simulink model "Basic_PLL_Beating1"  (R2014a)
settings: Solver=ode45  StartTime=0.0  StopTime=10.0  MaxStep=0.001  RelTol=1e-3
values from neighbouring files (symbols this model uses):
  IC_1 = 0.55    [Run_Basic_PLL_Beating1.m]
  IC_2 = -0.55    [Run_Basic_PLL_Beating1.m]
  Step_size = +0.47    (= 0.47)    [Run_Basic_PLL_Beating1.m]
settings Model: Creator=USER  LastModifiedBy=USER
settings SolverCC: InitialStep=0.001

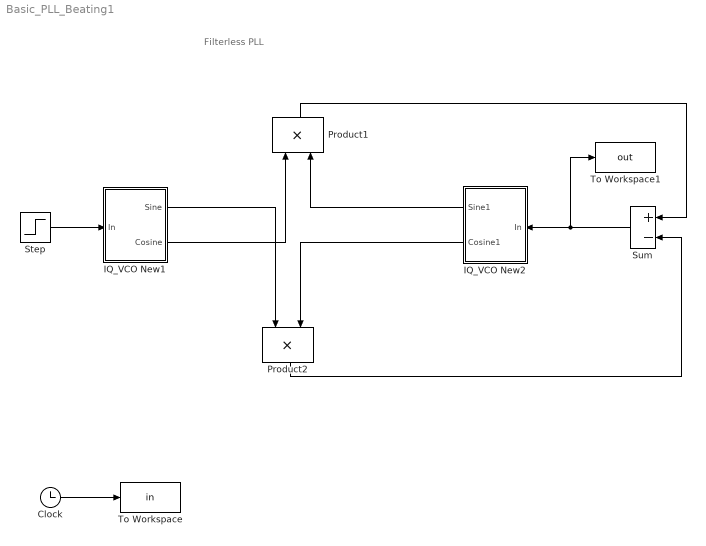
== system Basic_PLL_Beating1 ==
  note: Filterless PLL
  Clock : Clock
  IQ_VCO New1 : Subsystem
  IQ_VCO New2 : Subsystem
  Product1 : Product  SaturateOnIntegerOverflow=on  OutDataTypeStr=Inherit: Same as first input
  Product2 : Product  SaturateOnIntegerOverflow=on  OutDataTypeStr=Inherit: Same as first input
  Step : Step  Time=0  After=Step_size  SampleTime=0
  Sum : Sum  Inputs=+-  SaturateOnIntegerOverflow=on
  To Workspace : ToWorkspace  VariableName=in  SampleTime=-1
  To Workspace1 : ToWorkspace  VariableName=out  SampleTime=-1
  wires:
  Step/1 -> IQ_VCO New1/1(In)
  IQ_VCO New1/2(Cosine) -> Product1/1
  IQ_VCO New2/2(Cosine1) -> Product2/2
  IQ_VCO New1/1(Sine) -> Product2/1
  IQ_VCO New2/1(Sine1) -> Product1/2
  Sum/1 -> To Workspace1/1, IQ_VCO New2/1(In)
  Product1/1 -> Sum/1
  Product2/1 -> Sum/2
  Clock/1 -> To Workspace/1

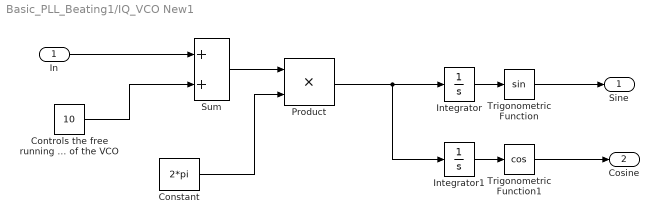
== system Basic_PLL_Beating1/IQ_VCO New1 ==
  In : Inport
  Constant : Constant  Value=2*pi
  "Controls the free running frequency (Hz) of the VCO " : Constant  Value=10
  Integrator : Integrator  InitialCondition=IC_1
  Integrator1 : Integrator  InitialCondition=IC_2
  Product : Product  SaturateOnIntegerOverflow=on  OutDataTypeStr=Inherit: Same as first input
  Sum : Sum  SaturateOnIntegerOverflow=on
  Trigonometric Function : Trigonometry
  Trigonometric Function1 : Trigonometry  Operator=cos
  Sine : Outport
  Cosine : Outport  Port=2
  wires:
  In/1 -> Sum/1
  "Controls the free running frequency (Hz) of the VCO "/1 -> Sum/2
  Sum/1 -> Product/1
  Constant/1 -> Product/2
  Trigonometric Function/1 -> Sine/1
  Trigonometric Function1/1 -> Cosine/1
  Integrator/1 -> Trigonometric Function/1
  Integrator1/1 -> Trigonometric Function1/1
  Product/1 -> Integrator1/1, Integrator/1

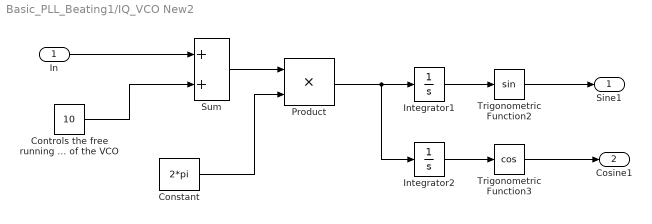
== system Basic_PLL_Beating1/IQ_VCO New2 ==
  In : Inport
  Constant : Constant  Value=2*pi
  "Controls the free running frequency (Hz) of the VCO " : Constant  Value=10
  Integrator1 : Integrator  InitialCondition=IC_1
  Integrator2 : Integrator  InitialCondition=IC_2
  Product : Product  SaturateOnIntegerOverflow=on  OutDataTypeStr=Inherit: Same as first input
  Sum : Sum  SaturateOnIntegerOverflow=on
  Trigonometric Function2 : Trigonometry
  Trigonometric Function3 : Trigonometry  Operator=cos
  Sine1 : Outport
  Cosine1 : Outport  Port=2
  wires:
  In/1 -> Sum/1
  "Controls the free running frequency (Hz) of the VCO "/1 -> Sum/2
  Sum/1 -> Product/1
  Constant/1 -> Product/2
  Trigonometric Function2/1 -> Sine1/1
  Trigonometric Function3/1 -> Cosine1/1
  Integrator1/1 -> Trigonometric Function2/1
  Integrator2/1 -> Trigonometric Function3/1
  Product/1 -> Integrator1/1, Integrator2/1
